simulink model "dspmrf_nhp"  (Simulink 5.0)
settings: Solver=FixedStepDiscrete  SolverMode=SingleTasking  StartTime=0.0  StopTime=inf  RelTol=1e-3  AbsTol=1e-6
PreLoadFcn:
  | load dspmrf_coeffs
undefined symbols (not defined in the file or in its folder): mrf_firdn1, mrf_upfir1
libraries: dspmlti3 x4, dspsrcs4 x1, dspmrf_lib x1
settings Model: Creator=don  LastModifiedBy=schim  ExtModeTrigMode=oneshot  ExtModeArmWhenConnect=off  SaveTime=off  SaveOutput=off  LimitDataPoints=off  IntegerOverflowMsg=none  BlockReductionOpt=off  BooleanDataType=off  RTWOptions=-aRollThreshold=2

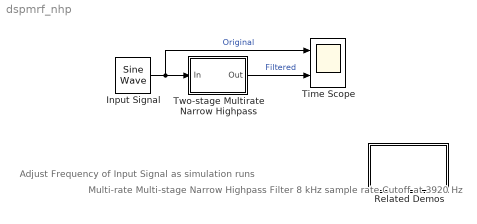
== system dspmrf_nhp ==
  note: Multi-rate Multi-stage
      | Narrow Highpass Filter
      |
      | 8 kHz sample rate
      | Cutoff at 3920 Hz
  note: Adjust Frequency
      | of Input Signal
      | as simulation runs
  Input Signal : dspsrcs4/Sine Wave  Amplitude=1  Frequency=4000-40  Phase=0  SampleMode=Discrete  OutComplex=Real  CompMethod=Trigonometric fcn  TableSize=Speed  SampleTime=1/8000  SamplesPerFrame=1  dataType=double  wordLen=16  udDataType=sfix(16)  fracBitsMode=Best precision  numFracBits=14  ResetState=Restart at time zero
  Related Demos : Subsystem
      settings: OpenFcn=dspmrf_menu
      mask Display: disp('Other\nMultirate Filter\nDemos')
  Time Scope : Scope  NumInputPorts=2
      settings: TimeRange=1.5  YMin=-1.5~-1.5  YMax=1.5~1.5  DataFormat=Structure
  Two-stage Multirate Narrow Highpass : Subsystem
  wires:
  Input Signal/1 -> Time Scope/1, Two-stage Multirate Narrow Highpass/1(In)  "Original"
  Two-stage Multirate Narrow Highpass/1(Out) -> Time Scope/2  "Filtered"

== system dspmrf_nhp/Related Demos ==

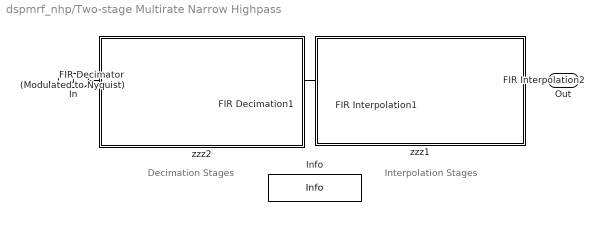
== system dspmrf_nhp/Two-stage Multirate Narrow Highpass ==
  note: Interpolation Stages
  note: Decimation Stages
  In : Inport
  FIR Decimation1 : dspmlti3/FIR Decimation  h=mrf_firdn2  D=4  framing=Maintain input frame size
  FIR Interpolation1 : dspmlti3/FIR Interpolation  h=mrf_upfir2  L=4  framing=Maintain input frame size
  FIR Interpolation2 : dspmlti3/FIR Interpolation  h=mrf_upfir1 .* ((-1).^(0:684))  L=12  framing=Maintain input frame size
  FIR Decimator (Modulated to Nyquist) : dspmlti3/FIR Decimation  h=mrf_firdn1 .* ((-1).^(0:684))  D=12  framing=Maintain input frame size
  Info : dspmrf_lib/Info
  zzz1 : Subsystem
      settings: OpenFcn=dspmsmrff;
      mask Display: disp('')
  zzz2 : Subsystem
      settings: OpenFcn=dspmsmrff;
      mask Display: disp('')
  Out : Outport
  wires:
  FIR Interpolation2/1 -> Out/1
  FIR Interpolation1/1 -> FIR Interpolation2/1
  FIR Decimation1/1 -> FIR Interpolation1/1
  FIR Decimator (Modulated to Nyquist)/1 -> FIR Decimation1/1
  In/1 -> FIR Decimator (Modulated to Nyquist)/1

== system dspmrf_nhp/Two-stage Multirate Narrow Highpass/zzz1 ==

== system dspmrf_nhp/Two-stage Multirate Narrow Highpass/zzz2 ==
